simulink model "noisySignal"  (R2015a)
settings: Solver=ode45  StartTime=0.0  StopTime=10.0  RelTol=1e-3
settings Model: Creator=John  LastModifiedBy=John

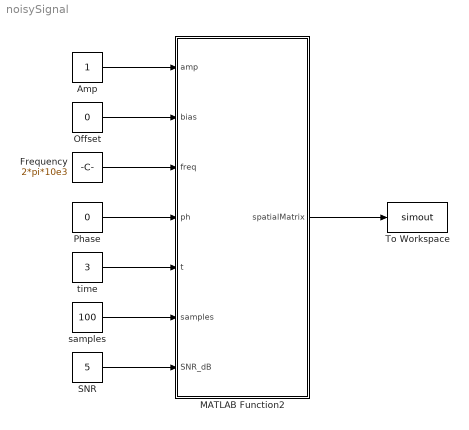
== system noisySignal ==
  Amp : Constant
  Frequency : Constant  Value=2*pi*10e3
  MATLAB Function2 : MATLAB Function  TreatAsAtomicUnit=on
  Offset : Constant  Value=0
  Phase : Constant  Value=0
  SNR : Constant  Value=5
  To Workspace : ToWorkspace  VariableName=simout  SaveFormat=Structure  SampleTime=-1
      settings: Save2DSignal=2-D array (concatenate along first dimension)
  samples : Constant  Value=100
  time : Constant  Value=3
  wires:
  Amp/1 -> MATLAB Function2/1(amp)
  Offset/1 -> MATLAB Function2/2(bias)
  Frequency/1 -> MATLAB Function2/3(freq)
  Phase/1 -> MATLAB Function2/4(ph)
  samples/1 -> MATLAB Function2/6(samples)
  time/1 -> MATLAB Function2/5(t)
  MATLAB Function2/1(spatialMatrix) -> To Workspace/1
  SNR/1 -> MATLAB Function2/7(SNR_dB)

== matlab function noisySignal/MATLAB Function2 ==
  data: amp input; spatialMatrix output size=[100,2]; bias input; freq input; ph input; t input; samples input; SNR_dB input
function spatialMatrix  = createSineWave(amp, bias, freq, ph, t, samples,SNR_dB)
% function spatialMatrix  = createSineWave(amp, bias, freq, ph, t, samples,SNR_dB)

%Variable Declaration
amplitude = amp; offset = bias;
frequency = freq; phase = ph;

time = linspace(0,t,samples);%Time Vector
outputWave = amplitude.*sin(frequency.*time + phase) + offset;

time = time'; outputWave = outputWave';
[noisyOutputWave, ~] = awgn(outputWave,SNR_dB);
spatialMatrix = cat(2,time,noisyOutputWave);
end
